simulink model "Light_Tracker"  (R2016b)
settings: Solver=FixedStepAuto  StartTime=0.0  StopTime=inf  RelTol=1e-3  EnableMultiTasking=on
libraries: arduinolib x5, simulink x1
settings Model: SimulationMode=external  ExtModeTrigDuration=2  Creator=Daniel  LastModifiedBy=Daniel
settings OptimizationCC: MaxStackSize=64
settings DebuggingCC: ParameterTunabilityLossMsg=error
settings HardwareCC: ProdBitPerInt=16  ProdBitPerPointer=16  ProdBitPerSizeT=16  ProdBitPerPtrDiffT=16  ProdLargestAtomicFloat=None  ProdWordSize=8  ProdHWDeviceType=Atmel->AVR  UseEmbeddedCoderFeatures=off  UseSimulinkCoderFeatures=off
settings RTWCC: SystemTargetFile=ert.tlc  HardwareBoard=Arduino Uno  TLCOptions=-aInlineSetEventsForThisBaseRateFcn=TLC_FALSE -aSuppressMultiTaskScheduler=TLC_FALSE -aRateBasedStepFcn=1  TemplateMakefile=ert_default_tmf  Description=Embedded Coder  GenerateReport=on  Toolchain=Arduino AVR v1.6.7  BuildConfiguration=Faster Runs  LaunchReport=on
settings CodeAppCC: ForceParamTrailComments=on  OperatorAnnotations=on  MATLABSourceComments=on
settings ERTTargetCC: ERTCustomFileBanners=off  SupportContinuousTime=on  SupportNonInlinedSFcns=on  RemoveResetFunc=off  SupportVariableSizeSignals=on  ModelStepFunctionPrototypeControlCompliant=off

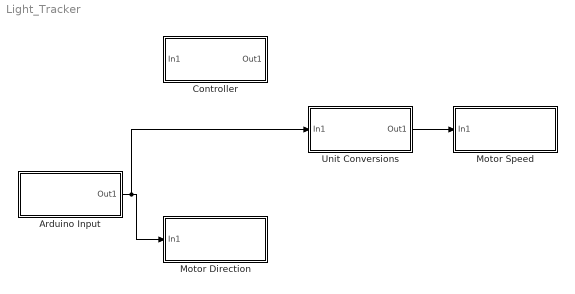
== system Light_Tracker ==
  Arduino Input : Subsystem
  Controller : Subsystem
  "Motor Direction " : Subsystem
  "Motor Speed " : Subsystem
  Unit Conversions : Subsystem
  wires:
  Unit Conversions/1(Out1) -> "Motor Speed "/1(In1)
  Arduino Input/1(Out1) -> Unit Conversions/1(In1), "Motor Direction "/1(In1)

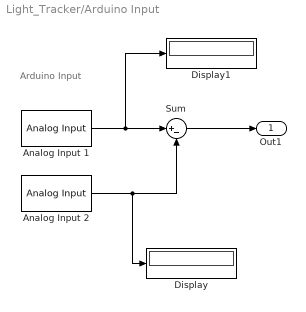
== system Light_Tracker/Arduino Input ==
  note: Arduino Input
  Analog Input 1 : arduinolib/Analog Input  pinNumber=4  sampleTime=.1  blockPlatform=arduino
  Analog Input 2 : arduinolib/Analog Input  pinNumber=5  sampleTime=.1  blockPlatform=arduino
  Display : Display
  Display1 : Display
  Sum : Sum  Inputs=|+-  OutDataTypeStr=double
  Out1 : Outport
  wires:
  Analog Input 2/1 -> Display/1, Sum/2
  Sum/1 -> Out1/1
  Analog Input 1/1 -> Display1/1, Sum/1

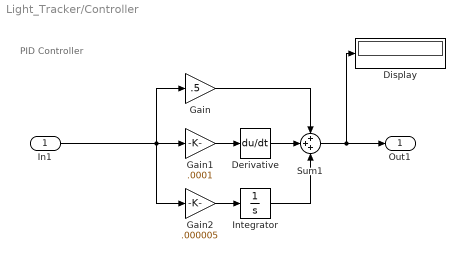
== system Light_Tracker/Controller ==
  note: PID Controller
  In1 : Inport
  Derivative : Derivative
  Display : Display
  Gain : Gain  Gain=.5
  Gain1 : Gain  Gain=.0001
  Gain2 : Gain  Gain=.000005
  Integrator : Integrator
  Sum1 : Sum  Inputs=+++
  Out1 : Outport
  wires:
  In1/1 -> Gain2/1, Gain1/1, Gain/1
  Gain1/1 -> Derivative/1
  Derivative/1 -> Sum1/2
  Gain/1 -> Sum1/1
  Sum1/1 -> Display/1, Out1/1
  Gain2/1 -> Integrator/1
  Integrator/1 -> Sum1/3

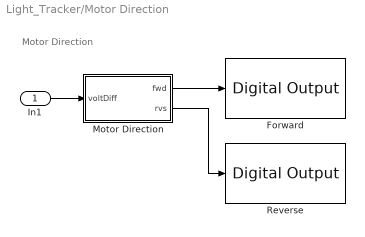
== system Light_Tracker/Motor Direction  ==
  note: Motor Direction
  In1 : Inport
  Forward : arduinolib/Digital Output  pinNumber=2  blockPlatform=arduino
  Motor Direction : MATLAB Function  TreatAsAtomicUnit=on
  Reverse : arduinolib/Digital Output  pinNumber=3  blockPlatform=arduino
  wires:
  Motor Direction/1(fwd) -> Forward/1
  Motor Direction/2(rvs) -> Reverse/1
  In1/1 -> Motor Direction/1(voltDiff)

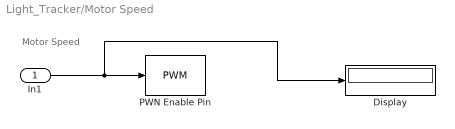
== system Light_Tracker/Motor Speed  ==
  note: Motor Speed
  In1 : Inport
  Display : Display
  PWN Enable Pin : arduinolib/PWM  pinNumber=9  blockPlatform=arduino
  wires:
  In1/1 -> Display/1, PWN Enable Pin/1

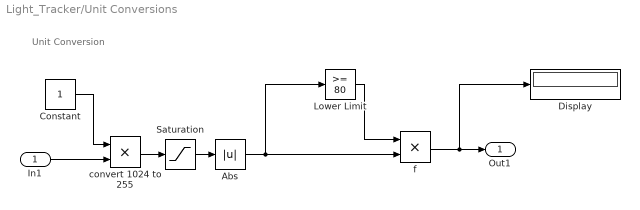
== system Light_Tracker/Unit Conversions ==
  note: Unit Conversion
  In1 : Inport
  Abs : Abs
  Constant : Constant
  Display : Display
  Lower Limit : simulink/Logic and Bit Operations/Compare To Constant  relop=>=  const=80  OutDataTypeStr=boolean
  Saturation : Saturate  UpperLimit=254  LowerLimit=-254
  convert 1024 to 255 : Product
  f : Product
  Out1 : Outport
  wires:
  In1/1 -> convert 1024 to 255/2
  Constant/1 -> convert 1024 to 255/1
  convert 1024 to 255/1 -> Saturation/1
  Abs/1 -> Lower Limit/1, f/2
  Lower Limit/1 -> f/1
  f/1 -> Display/1, Out1/1
  Saturation/1 -> Abs/1

== matlab function Light_Tracker/Motor Direction /Motor Direction ==
  data: voltDiff input; fwd output; rvs output
function [fwd,rvs] = fcn(voltDiff)


if voltDiff > 0 
    fwd = 1; % motor forward
    rvs = 0;

else
    fwd = 0; % motor reverse
    rvs = 1; 

end
